simulink model "SIMU"  (R2015b)
settings: Solver=VariableStepAuto  StartTime=0.0  StopTime=P1((length(P1)),1)  RelTol=1e-3
libraries: arduino_io_lib x11, simulink x3
settings Model: Creator=Alvaro  LastModifiedBy=Alvaro
settings OptimizationCC: BlockReduction=off  DefaultParameterBehavior=Inlined
settings HardwareCC: ProdBitPerInt=16  ProdBitPerPointer=16  ProdLargestAtomicFloat=None  ProdWordSize=8  ProdHWDeviceType=Atmel->AVR

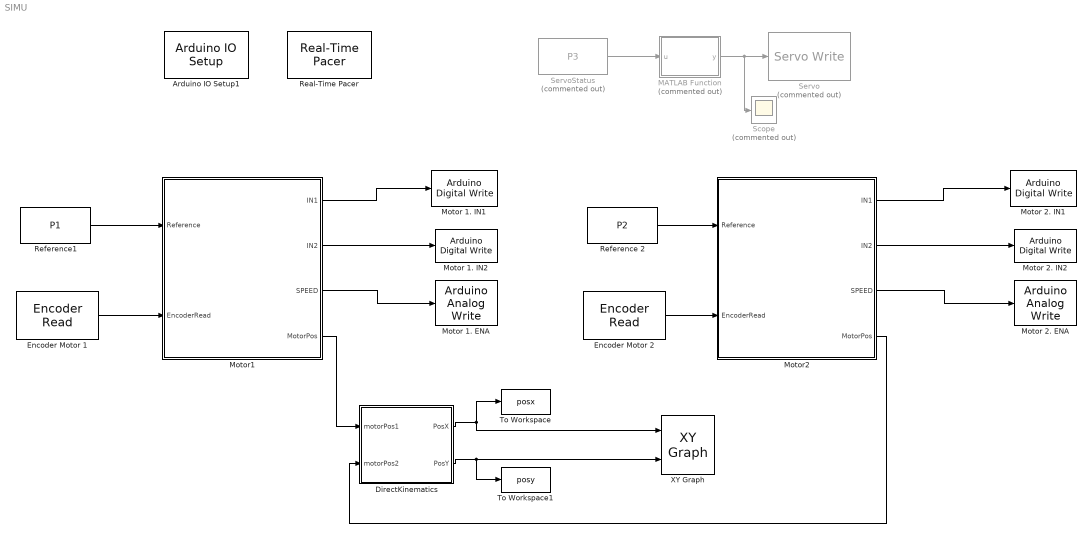
== system SIMU ==
  Arduino IO Setup1 : arduino_io_lib/Arduino IO Setup  Priority=3  arduinoVar=Temporary arduino variable: Arduino1  workspaceVarName=a  comPort=COM6
      settings: AttributesFormatString=%<comPort>
  "DirectKinematics " : MATLAB Function  TreatAsAtomicUnit=on
  "Encoder Motor 1 " : arduino_io_lib/Encoder Read  arduinoVar=Temporary arduino variable: Arduino1  encNum=0  pinA=2  pinB=3  DbDl=0  T=0.01
  "Encoder Motor 2 " : arduino_io_lib/Encoder Read  arduinoVar=Temporary arduino variable: Arduino1  encNum=1  pinA=19  pinB=18  DbDl=0  T=0.01
  MATLAB Function : MATLAB Function  Commented=on  TreatAsAtomicUnit=on
  "Motor 1. ENA " : arduino_io_lib/Arduino Analog Write  arduinoVar=Temporary arduino variable: Arduino1  arduinoPin=7  T=0.01
  Motor 1. IN1 : arduino_io_lib/Arduino Digital Write  arduinoVar=Temporary arduino variable: Arduino1  arduinoPin=5  T=0.01
  Motor 1. IN2 : arduino_io_lib/Arduino Digital Write  arduinoVar=Temporary arduino variable: Arduino1  arduinoPin=6  T=0.01
  "Motor 2. ENA " : arduino_io_lib/Arduino Analog Write  arduinoVar=Temporary arduino variable: Arduino1  arduinoPin=10  T=0.01
  "Motor 2. IN1 " : arduino_io_lib/Arduino Digital Write  arduinoVar=Temporary arduino variable: Arduino1  arduinoPin=8  T=0.01
  "Motor 2. IN2 " : arduino_io_lib/Arduino Digital Write  arduinoVar=Temporary arduino variable: Arduino1  arduinoPin=9  T=0.01
  "Motor1 " : Subsystem
  "Motor2 " : Subsystem
  Real-Time Pacer : arduino_io_lib/Real-Time Pacer  simTimePerRealTime=0.88
  "Reference 2 " : FromWorkspace  VariableName=P2  SampleTime=0.01
  "Reference1 " : FromWorkspace  VariableName=P1  SampleTime=0.01
  Scope : Scope  Commented=on
  Servo : arduino_io_lib/Servo Write  Commented=on  arduinoVar=Temporary arduino variable: Arduino1  pinNum=46  T=0.01
  "ServoStatus " : FromWorkspace  Commented=on  VariableName=P3  SampleTime=0.01
  To Workspace : ToWorkspace  VariableName=posx  SaveFormat=Timeseries  SampleTime=0.01
      settings: Decimation=4
  To Workspace1 : ToWorkspace  VariableName=posy  SaveFormat=Timeseries  SampleTime=0.01
  XY Graph : simulink/Sinks/XY Graph  xmin=-15  xmax=15  ymin=0  ymax=21  st=0.01
  wires:
  "Motor1 "/3("SPEED ") -> "Motor 1. ENA "/1
  "Motor1 "/2("IN2 ") -> Motor 1. IN2/1
  "Reference1 "/1 -> "Motor1 "/1(Reference)
  "Encoder Motor 1 "/1 -> "Motor1 "/2("EncoderRead ")
  "Motor1 "/1(IN1) -> Motor 1. IN1/1
  "Motor2 "/3("SPEED ") -> "Motor 2. ENA "/1
  "Motor2 "/2("IN2 ") -> "Motor 2. IN2 "/1
  "Reference 2 "/1 -> "Motor2 "/1(Reference)
  "Encoder Motor 2 "/1 -> "Motor2 "/2("EncoderRead ")
  "Motor2 "/1(IN1) -> "Motor 2. IN1 "/1
  "Motor1 "/4(MotorPos) -> "DirectKinematics "/1(motorPos1)
  "DirectKinematics "/1(PosX) -> To Workspace/1, XY Graph/1
  "DirectKinematics "/2(PosY) -> To Workspace1/1, XY Graph/2
  "Motor2 "/4(MotorPos) -> "DirectKinematics "/2(motorPos2)
  "ServoStatus "/1 -> MATLAB Function/1(u)
  MATLAB Function/1(y) -> Scope/1, Servo/1

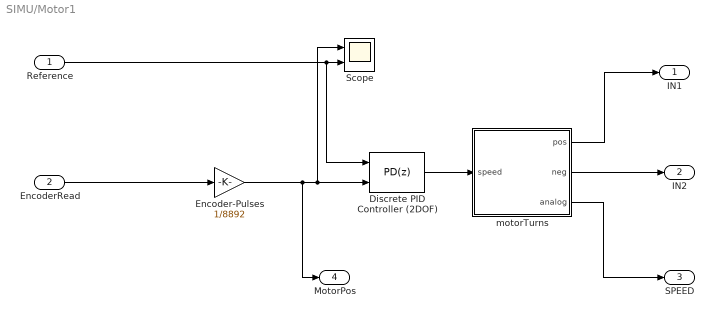
== system SIMU/Motor1  ==
  Reference : Inport
  "EncoderRead " : Inport  Port=2
  Discrete PID Controller (2DOF) : simulink/Continuous/PID Controller (2DOF)  Controller=PD  TimeDomain=Discrete-time  SampleTime=-1  IntegratorMethod=Forward Euler  FilterMethod=Forward Euler  Form=Parallel  UseFilter=on  ControllerParametersSource=internal  P=1600  I=1  D=2.5  N=10  b=1  c=1  InitialConditionSource=internal  InitialConditionForIntegrator=0  InitialConditionForFilter=0  ExternalReset=none  LimitOutput=on  UpperSaturationLimit=255  LowerSaturationLimit=-255  LinearizeAsGain=off  AntiWindupMode=none  Kb=1  TrackingMode=off  Kt=1  PParamMin=[]  PParamMax=[]  IParamMin=[]  IParamMax=[]  DParamMin=[]  DParamMax=[]  NParamMin=[]  NParamMax=[]  bParamMin=[]  bParamMax=[]  cParamMin=[]  cParamMax=[]  KbParamMin=[]  KbParamMax=[]  KtParamMin=[]  KtParamMax=[]  POutMin=[]  POutMax=[]  IOutMin=[]  IOutMax=[]  DOutMin=[]  DOutMax=[]  NOutMin=[]  NOutMax=[]  bOutMin=[]  bOutMax=[]  cOutMin=[]  cOutMax=[]  KbOutMin=[]  KbOutMax=[]  KtOutMin=[]  KtOutMax=[]  IntegratorOutMin=[]  IntegratorOutMax=[]  FilterOutMin=[]  FilterOutMax=[]  SumOutMin=[]  SumOutMax=[]  Sum1OutMin=[]  Sum1OutMax=[]  Sum2OutMin=[]  Sum2OutMax=[]  Sum3OutMin=[]  Sum3OutMax=[]  SumI1OutMin=[]  SumI1OutMax=[]  SumI2OutMin=[]  SumI2OutMax=[]  SumI3OutMin=[]  SumI3OutMax=[]  SumDOutMin=[]  SumDOutMax=[]  SaturationOutMin=[]  SaturationOutMax=[]  IntegratorContinuousStateAttributes=''  IntegratorStateMustResolveToSignalObject=off  IntegratorRTWStateStorageClass=Auto  FilterContinuousStateAttributes=''  FilterStateMustResolveToSignalObject=off  FilterRTWStateStorageClass=Auto  DifferentiatorICPrevScaledInput=0  DifferentiatorOutMin=[]  DifferentiatorOutMax=[]
  "Encoder-Pulses " : Gain  Gain=1/8892
  Scope : Scope  NumInputPorts=2
  "motorTurns " : MATLAB Function  TreatAsAtomicUnit=on
  IN1 : Outport
  "IN2 " : Outport  Port=2
  "SPEED " : Outport  Port=3
  MotorPos : Outport  Port=4
  wires:
  "motorTurns "/2(neg) -> "IN2 "/1
  "motorTurns "/1(pos) -> IN1/1
  "EncoderRead "/1 -> "Encoder-Pulses "/1
  Discrete PID Controller (2DOF)/1 -> "motorTurns "/1(speed)
  "motorTurns "/3(analog) -> "SPEED "/1
  Reference/1 -> Discrete PID Controller (2DOF)/1, Scope/2
  "Encoder-Pulses "/1 -> MotorPos/1, Discrete PID Controller (2DOF)/2, Scope/1

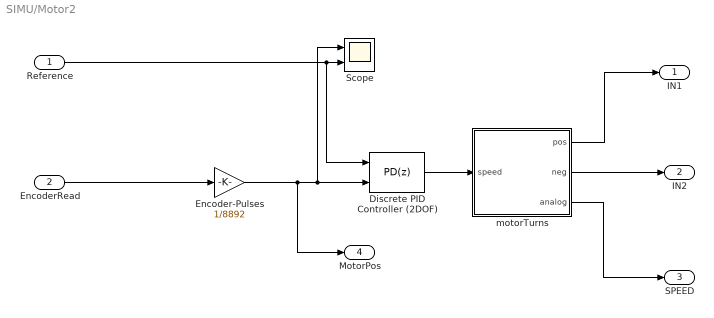
== system SIMU/Motor2  ==
  Reference : Inport
  "EncoderRead " : Inport  Port=2
  Discrete PID Controller (2DOF) : simulink/Continuous/PID Controller (2DOF)  Controller=PD  TimeDomain=Discrete-time  SampleTime=-1  IntegratorMethod=Forward Euler  FilterMethod=Forward Euler  Form=Parallel  UseFilter=on  ControllerParametersSource=internal  P=1600  I=1  D=2.5  N=10  b=1  c=1  InitialConditionSource=internal  InitialConditionForIntegrator=0  InitialConditionForFilter=0  ExternalReset=none  LimitOutput=on  UpperSaturationLimit=255  LowerSaturationLimit=-255  LinearizeAsGain=off  AntiWindupMode=none  Kb=1  TrackingMode=off  Kt=1  PParamMin=[]  PParamMax=[]  IParamMin=[]  IParamMax=[]  DParamMin=[]  DParamMax=[]  NParamMin=[]  NParamMax=[]  bParamMin=[]  bParamMax=[]  cParamMin=[]  cParamMax=[]  KbParamMin=[]  KbParamMax=[]  KtParamMin=[]  KtParamMax=[]  POutMin=[]  POutMax=[]  IOutMin=[]  IOutMax=[]  DOutMin=[]  DOutMax=[]  NOutMin=[]  NOutMax=[]  bOutMin=[]  bOutMax=[]  cOutMin=[]  cOutMax=[]  KbOutMin=[]  KbOutMax=[]  KtOutMin=[]  KtOutMax=[]  IntegratorOutMin=[]  IntegratorOutMax=[]  FilterOutMin=[]  FilterOutMax=[]  SumOutMin=[]  SumOutMax=[]  Sum1OutMin=[]  Sum1OutMax=[]  Sum2OutMin=[]  Sum2OutMax=[]  Sum3OutMin=[]  Sum3OutMax=[]  SumI1OutMin=[]  SumI1OutMax=[]  SumI2OutMin=[]  SumI2OutMax=[]  SumI3OutMin=[]  SumI3OutMax=[]  SumDOutMin=[]  SumDOutMax=[]  SaturationOutMin=[]  SaturationOutMax=[]  IntegratorContinuousStateAttributes=''  IntegratorStateMustResolveToSignalObject=off  IntegratorRTWStateStorageClass=Auto  FilterContinuousStateAttributes=''  FilterStateMustResolveToSignalObject=off  FilterRTWStateStorageClass=Auto  DifferentiatorICPrevScaledInput=0  DifferentiatorOutMin=[]  DifferentiatorOutMax=[]
  "Encoder-Pulses " : Gain  Gain=1/8892
  Scope : Scope  NumInputPorts=2
  "motorTurns " : MATLAB Function  TreatAsAtomicUnit=on
  IN1 : Outport
  "IN2 " : Outport  Port=2
  "SPEED " : Outport  Port=3
  MotorPos : Outport  Port=4
  wires:
  "motorTurns "/2(neg) -> "IN2 "/1
  "Encoder-Pulses "/1 -> MotorPos/1, Discrete PID Controller (2DOF)/2, Scope/1
  "motorTurns "/1(pos) -> IN1/1
  "EncoderRead "/1 -> "Encoder-Pulses "/1
  Discrete PID Controller (2DOF)/1 -> "motorTurns "/1(speed)
  "motorTurns "/3(analog) -> "SPEED "/1
  Reference/1 -> Discrete PID Controller (2DOF)/1, Scope/2

== matlab function SIMU/Motor2 /motorTurns  ==
  data: speed input; pos output; neg output; analog output
function [pos,neg,analog] = motorTurns(speed)

if (speed>0)
    pos=1;
    neg=0;
    analog=speed;
elseif (speed<0)
    pos=0;
    neg=1;
    analog=-speed;
else
    pos=0;
    neg=0;
    analog=0;
end
    
end

== matlab function SIMU/DirectKinematics  ==
  data: motorPos1 input; motorPos2 input; PosX output; PosY output
function [PosX,PosY] = fcn(motorPos1,motorPos2)
L=33.5005;
RR=1.8;
RP=0.6;
PosX=2*pi*RP*motorPos2*sin(atan((2*pi*RR*motorPos1)/L));
PosY=2*pi*RP*motorPos2*cos(atan((2*pi*RR*motorPos1)/L));
end

== matlab function SIMU/Motor1 /motorTurns  ==
  data: speed input; pos output; neg output; analog output
function [pos,neg,analog] = motorTurns(speed)

if (speed>0)
    pos=1;
    neg=0;
    analog=speed;
elseif (speed<0)
    pos=0;
    neg=1;
    analog=-speed;
else
    pos=0;
    neg=0;
    analog=0;
end
    
end

== matlab function SIMU/MATLAB Function ==
  data: u input; y output
function y = fcn(u)
if(u==1)
    y=68;
else
    y=80;
end
end
